simulink model "Ne_proj_zad1"  (R2022b)
settings: Solver=ode3  StartTime=0.0  StopTime=0.3  FixedStep=1e-4  RelTol=1e-3
values from neighbouring files (symbols this model uses):
  B = J*Rt/(fie^2)    (= 0.0343267040258)    [NE_proj_zad2.m]
  Rt = 0.254    [NE_proj_zad2.m]
  T = 0.001*Lt/Rt    (= 0.00641732283465)    [NE_proj_zad2.m]
  UN = 440    [NE_proj_zad2.m]
undefined symbols (not defined in the file or in its folder): psie
settings Model: Creator=womru  LastModifiedBy=womru
settings DataIOCC: SaveFormat=StructureWithTime  ReturnWorkspaceOutputs=off
settings OptimizationCC: ReuseModelBlockBuffer=on

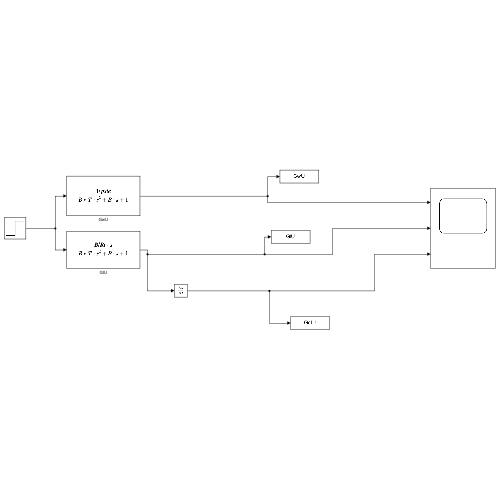
[thumbnail: Simulink's stored preview of the top-level diagram]
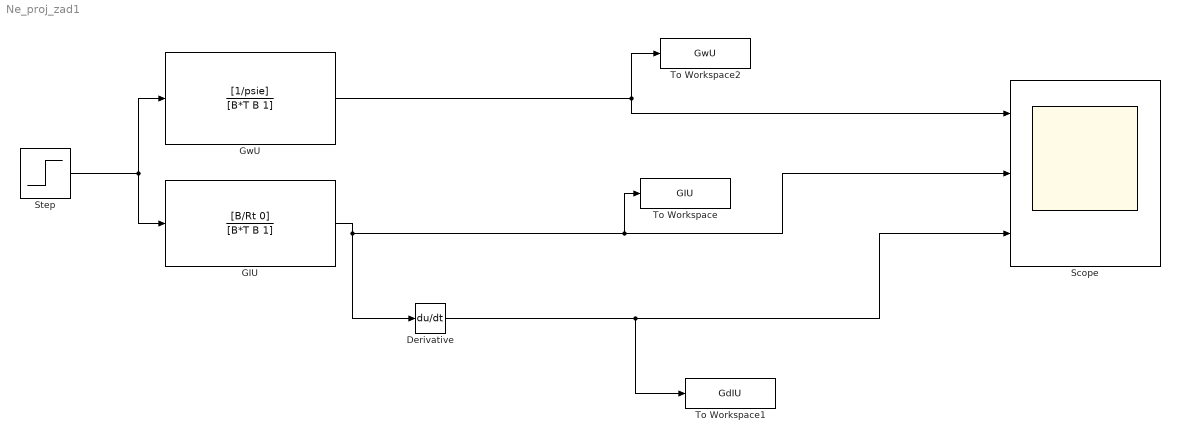
== system Ne_proj_zad1 ==
  Derivative : Derivative
  GIU : TransferFcn  Numerator=[B/Rt 0]  Denominator=[B*T B 1]
  GwU : TransferFcn  Numerator=[1/psie]  Denominator=[B*T B 1]
  Scope : Scope  NumInputPorts=3
  Step : Step  Time=0  After=UN  SampleTime=0
  To Workspace : ToWorkspace  VariableName=GIU  SaveFormat=Structure With Time  SampleTime=-1
  To Workspace1 : ToWorkspace  VariableName=GdIU  SaveFormat=Structure With Time  SampleTime=-1
  To Workspace2 : ToWorkspace  VariableName=GwU  SaveFormat=Structure With Time  SampleTime=-1
  wires:
  Step/1 -> GIU/1, GwU/1
  GwU/1 -> To Workspace2/1, Scope/1
  GIU/1 -> To Workspace/1, Scope/2, Derivative/1
  Derivative/1 -> To Workspace1/1, Scope/3
